simulink model "model_Tp0c"  (R2021a)
settings: Solver=ode45  StartTime=0.0  StopTime=5  MaxStep=1e-3  RelTol=1e-3
values from neighbouring files (symbols this model uses):
  J = (Tm*KN^2)/Ra    (= 0.00790540540541)    [Tp0.m]
  KN = Kt    (= 0.5)    [Tp0.m]
  Kpn = KN*(TM/(2*Ta)-1)    (= 0.222222222222)    [Tp0.m]
  La = Te*Ra    (= 0.0014985)    [Tp0.m]
  Ra = 0.37    [Tp0.m]
  Tc = 15    [Tp0.m]
  Tin = 4*Ta*(1-2*Ta/(TM))    (= 0.00498461538462)    [Tp0.m]
  wref = 392    [Tp0.m]
undefined symbols (not defined in the file or in its folder): b
libraries: simulink x2, pid_lib x1
settings Model: Creator=Lac User  LastModifiedBy=Windows
settings SolverCC: AlgebraicLoopSolver=TrustRegion
settings DataIOCC: SaveFormat=StructureWithTime
settings OptimizationCC: LifeSpan=inf
settings DebuggingCC: SFExecutionAtInitializationDiag=none  SFMachineParentedDataDiag=warning  ArithmeticOperatorsInVariantConditions=warning
settings HardwareCC: ProdBitPerSizeT=32  ProdBitPerPtrDiffT=32  ProdWordSize=32  ProdHWDeviceType=Specified
settings SFSimCC: CustomCodeUndefinedFunction=UseInterfaceOnly
settings CodeAppCC: StateflowObjectComments=on

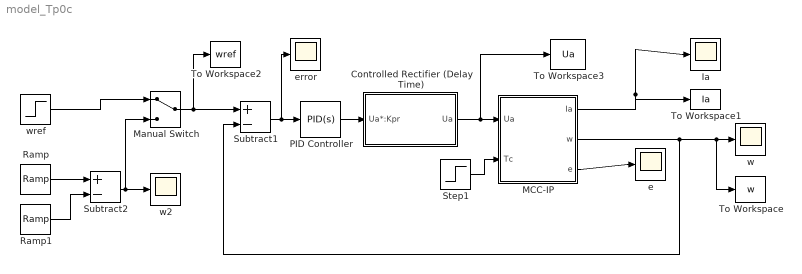
== system model_Tp0c ==
  Controlled Rectifier (Delay Time) : Subsystem  mask(Controlled Rectifier (Delay Time)){Tpr=0.2e-2, Kpr=1}
      mask prompts: Tpr "Delay Time:"; Kpr "Controlled Rectifier Proportional Gain:"
      mask help: Kpr.e(-Tpr.s)
      mask Display:
      | plot([0.5 0.6 0.6 0.75],[0.2 0.2 .8 .8 ])
      | plot([0.45 0.8 0.8 0.45 0.45],[0.15 0.15 .85 .85 0.15])
  Ia : Scope
  MCC-IP : Subsystem
  Manual Switch : ManualSwitch
  PID Controller : pid_lib/PID Controller  Controller=PID  Form=Parallel  TimeDomain=Continuous-time  UseExternalTs=off  SampleTime=-1  IntegratorMethod=Forward Euler  FilterMethod=Forward Euler  ControllerParametersSource=internal  P=Kpn  I=Kpn/Tin  D=0  UseFilter=on  N=100  TunerSelectOption=Transfer Function Based (PID Tuner App)  InitialConditionSource=internal  InitialConditionForIntegrator=0  InitialConditionForFilter=0  DifferentiatorICPrevScaledInput=0  ExternalReset=none  TrackingMode=off  Kt=1  LimitOutput=off  SatLimitsSource=internal  UpperSaturationLimit=inf  LowerSaturationLimit=-inf  LinearizeAsGain=on  AntiWindupMode=none  Kb=1  POutMin=[]  POutMax=[]  IOutMin=[]  IOutMax=[]  DOutMin=[]  DOutMax=[]  NOutMin=[]  NOutMax=[]  SumOutMin=[]  SumOutMax=[]  SaturationOutMin=[]  SaturationOutMax=[]  PParamMin=[]  PParamMax=[]  IParamMin=[]  IParamMax=[]  DParamMin=[]  DParamMax=[]  NParamMin=[]  NParamMax=[]  KbParamMin=[]  KbParamMax=[]  KtParamMin=[]  KtParamMax=[]  KbOutMin=[]  KbOutMax=[]  KtOutMin=[]  KtOutMax=[]  IntegratorOutMin=[]  IntegratorOutMax=[]  FilterOutMin=[]  FilterOutMax=[]  SumI1OutMin=[]  SumI1OutMax=[]  SumI2OutMin=[]  SumI2OutMax=[]  SumI3OutMin=[]  SumI3OutMax=[]  SumI4OutMin=[]  SumI4OutMax=[]  SumDOutMin=[]  SumDOutMax=[]  DifferentiatorOutMin=[]  DifferentiatorOutMax=[]  FilterDiffOutCoefMin=[]  FilterDiffOutCoefMax=[]  ReciprocalOutMin=[]  ReciprocalOutMax=[]  SumDenOutMin=[]  SumDenOutMax=[]  SumNumOutMin=[]  SumNumOutMax=[]  DivideOutMin=[]  DivideOutMax=[]  UdiffTsProdOutMin=[]  UdiffTsProdOutMax=[]  NTsProdOutMin=[]  NTsProdOutMax=[]  UintegralTsProdOutMin=[]  UintegralTsProdOutMax=[]  UngainTsProdOutMin=[]  UngainTsProdOutMax=[]  IntegratorContinuousStateAttributes=''  IntegratorStateMustResolveToSignalObject=off  IntegratorRTWStateStorageClass=Auto  FilterContinuousStateAttributes=''  FilterStateMustResolveToSignalObject=off  FilterRTWStateStorageClass=Auto  ParallelPVariant=InternalParameters  IdealPVariant=Disabled  IVariant=InternalParameters  DVariant=InternalParameters  IntegratorVariant=Continuous  SatVariant=Disabled  AWVariant=Passthrough  PCopyVariant=Disabled  TRVariant=Disabled  FdbkBlocksVariant=Forward  IdealPFdbkVariant=Disabled  SatFdbkVariant=Disabled  DerivativeFilterVariant=ContFilter  NVariant=InternalParameters  NCopyVariant=Disabled  FilterICVariant=InternalICsFilter  IntegratorICVariant=InternalICs  ExternalResetVariant=Disabled  TRSumVariant=Passthrough  SumFdbkVariant=Disabled  SumVariant=Sum_PID  TsampFilterVariant=InternalTs  TsampNgainVariant=Passthrough  TsampIntegralVariant=Passthrough  ExternalSaturationOutDataTypeStr=Inherit: Same as second input
  Ramp : simulink/Sources/Ramp  slope=wref*4  start=0  InitialOutput=0
  Ramp1 : simulink/Sources/Ramp  slope=wref*4  start=0.25  InitialOutput=0
  Step1 : Step  Time=2.5  After=Tc  SampleTime=0
  Subtract1 : Sum  Inputs=+-
  Subtract2 : Sum  Inputs=+-
  To Workspace : ToWorkspace  VariableName=w  SampleTime=-1
  To Workspace1 : ToWorkspace  VariableName=Ia  SampleTime=-1
  To Workspace2 : ToWorkspace  VariableName=wref  SampleTime=-1
  To Workspace3 : ToWorkspace  VariableName=Ua  SampleTime=-1
  e : Scope
  error : Scope
  w : Scope
  w2 : Scope
  wref : Step  Time=0  After=wref  SampleTime=0
  wires:
  MCC-IP/1(Ia) -> To Workspace1/1, Ia/1
  MCC-IP/3(e) -> e/1
  Subtract1/1 -> error/1, PID Controller/1
  Step1/1 -> MCC-IP/2(Tc)
  Subtract2/1 -> Manual Switch/2, w2/1
  Ramp/1 -> Subtract2/1
  Ramp1/1 -> Subtract2/2
  wref/1 -> Manual Switch/1
  Manual Switch/1 -> To Workspace2/1, Subtract1/1
  PID Controller/1 -> Controlled Rectifier (Delay Time)/1(Ua*:Kpr)
  Controlled Rectifier (Delay Time)/1(Ua) -> To Workspace3/1, MCC-IP/1(Ua)
  MCC-IP/2(w) -> Subtract1/2, To Workspace/1, w/1

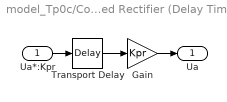
== system model_Tp0c/Controlled Rectifier (Delay Time) ==
  Ua*:Kpr : Inport
  Gain : Gain  Gain=Kpr  SaturateOnIntegerOverflow=on  OutDataTypeStr=Inherit: Same as input  ParamDataTypeStr=Inherit: Same as input
  Transport Delay : TransportDelay  DelayTime=Tpr
  Ua : Outport  VectorParamsAs1DForOutWhenUnconnected=off
  wires:
  Gain/1 -> Ua/1
  Transport Delay/1 -> Gain/1
  Ua*:Kpr/1 -> Transport Delay/1

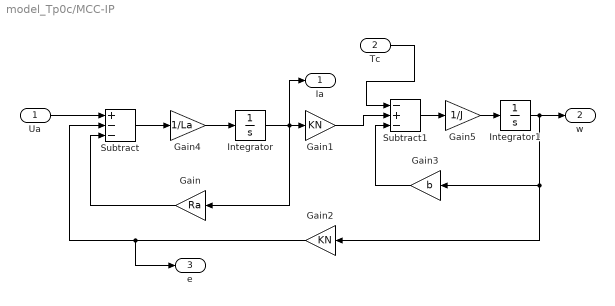
== system model_Tp0c/MCC-IP ==
  Ua : Inport
  Tc : Inport  Port=2
  Gain : Gain  Gain=Ra
  Gain1 : Gain  Gain=KN
  Gain2 : Gain  Gain=KN
  Gain3 : Gain  Gain=b
  Gain4 : Gain  Gain=1/La
  Gain5 : Gain  Gain=1/J
  Integrator : Integrator
  Integrator1 : Integrator
  Subtract : Sum  Inputs=+--
  Subtract1 : Sum  Inputs=-+-
  Ia : Outport  VectorParamsAs1DForOutWhenUnconnected=off
  w : Outport  Port=2  VectorParamsAs1DForOutWhenUnconnected=off
  e : Outport  Port=3  VectorParamsAs1DForOutWhenUnconnected=off
  wires:
  Subtract1/1 -> Gain5/1
  Gain4/1 -> Integrator/1
  Gain1/1 -> Subtract1/2
  Subtract/1 -> Gain4/1
  Integrator1/1 -> Gain3/1, Gain2/1, w/1
  Integrator/1 -> Ia/1, Gain/1, Gain1/1
  Gain2/1 -> e/1, Subtract/2
  Gain/1 -> Subtract/3
  Gain5/1 -> Integrator1/1
  Ua/1 -> Subtract/1
  Tc/1 -> Subtract1/1
  Gain3/1 -> Subtract1/3
